simulink model "a01_SimTurret"  (R2024a)
settings: Solver=VariableStepAuto  StartTime=0.0  StopTime=10  FixedStep=0.000001  MaxStep=mSim.dTime*0.01  RelTol=mSim.dTime*0.01
PostLoadFcn:
  | a02_SimVariable
undefined symbols (not defined in the file): A02MTRPA, a1st, B01SCHED, b5th, C01ISENS, c7th, CRX1, DC, E03LIM, H01MDE, H01TRT, Init, mDefine, Mech, mSim, MtrPar, Sim, SIM, SimMde
libraries: spsSeriesRLCBranchLib x17, simulink x8, spsCurrentMeasurementLib x7, spsIGBTDiodeLib x7, spsDiodeLib x6, spsControlledVoltageSourceLib x6, spsVoltageMeasurementLib x4, SignalEditorBlockLib x3, spsDCVoltageSourceLib x1, spspowerguiLib x1
(part 3 of 3)

== stateflow chart a01_SimTurret/ASW_Composition/Subsystem/Nftn_StateManagement/Chart_StateManagement ==
  state Normal
    entry:
    mSMDE_uFlagRestart = Cnst_u16False;
    during:
    Ftn_CalActAngle();
    state Ftn_CalActAngle [function]
      (default) -> (junction 265) : // Calculation Acture Angle
      (junction 265) -> (junction 326) : {
          | sTemp = single(mMTPST_i64TurretPst - mSMDE_i64PstOrigin);
          | sTemp = sTemp * sAngleTrGain;
          | }
      (junction 326) -> (junction 328) [order 1] : [sTemp > Cnst_sZero]
      (junction 326) -> (junction 329) [order 2] : {
          | sTemp = (sTemp - single(int16(sTemp * Cnst_sInv360) * Cnst_s360)) + Cnst_s360;
          | }
      (junction 328) -> (junction 331) : {
          | sTemp = sTemp - single(int16(sTemp * Cnst_sInv360) * Cnst_s360);
          | }
      (junction 331) -> (junction 329)
      (junction 329) -> (junction 314)
      (junction 314) -> (junction 315) [order 1] : [sTemp > Cnst_s360]
      (junction 314) -> (junction 319) [order 2]
      (junction 315) -> (junction 317) : {
          | sTemp = sTemp - Cnst_s360;
          | }
      (junction 319) -> (junction 321) [order 1] : [sTemp < Cnst_sZero]
      (junction 319) -> (junction 316) [order 2] : {
          | sTemp = sTemp;
          | }
      (junction 321) -> (junction 322) : {
          | sTemp = sTemp + Cnst_s360;
          | }
      (junction 322) -> (junction 316)
      (junction 317) -> (junction 322)
      (junction 316) -> (junction 346)
      (junction 346) -> (junction 347) [order 1] : [uTurretDirection == Cnst_u16True]
      (junction 346) -> (junction 348) [order 2] : {
          | mSMDE_sActAngle = sTemp;
          | }
      (junction 347) -> (junction 349) : {
          | mSMDE_sActAngle = Cnst_s360 - sTemp;
          | }
      (junction 349) -> (junction 348)
      (junction 348) -> (junction 1542)
      (junction 1542) -> (junction 1543) [order 1] : [mSMDE_sRefAngle < Cnst_sZero]
      (junction 1543) -> (junction 1545) : {
          | mSMDE_sRefAngleDisp = mSMDE_sRefAngle + Cnst_s360;
          | }
      (junction 1542) -> (junction 1544) [order 2] : {
          | mSMDE_sRefAngleDisp = mSMDE_sRefAngle;
          | }
      (junction 1545) -> (junction 1544)
      (junction 1544) -> (junction 1546)
    note: 현재 위치 계산
    state Ftn_CalRefAngle [function]
      (default) -> (junction 799) : // Calculation Reference Angle
      (junction 799) -> (junction 896) [order 1] : [(mSMDE_i64PstOrigin ~= 0)&&(mCRX_uRefPst >= Cnst_u16One)]
      (junction 896) -> (junction 897)
      (junction 799) -> (junction 805) [order 2] : {
          | // Index 0 is not a valid value, but if index 0 is received, it is configured to move to the origin.
          | mSMDE_sRefAngle = Cnst_sZero;
          | }
      (junction 897) -> (junction 800) [order 1] : [(mCRX_uStart == Cnst_u16True)&&(uStartZ == Cnst_u16False)]
      (junction 897) -> (junction 900) [order 2] : // No Action
      (junction 800) -> (junction 801) : {
          | uFlagJogMde = Cnst_u16False;
          | }
      (junction 801) -> (junction 802) [order 1] : [mCRX_uRefPst > u16NumOfTool]
      (junction 801) -> (junction 803) [order 2] : {
          | uRefPst = mCRX_uRefPst;
          | }
      (junction 802) -> (junction 804) : {
          | uRefPst = u16NumOfTool;
          | }
      (junction 804) -> (junction 803)
      (junction 803) -> (junction 806) : {
          | mSMDE_sRefAngle = (single(uRefPst - Cnst_u16One) * sAnglePerTool);
          | Ftn_CalRefPst();
          | }
      (junction 806) -> (junction 900)
      (junction 900) -> (junction 805)
      (junction 805) -> (junction 807) : {
          | uStartZ = mCRX_uStart;
          | }
    note: Start 신호 입력시 Ref Angle 계산
    state Ftn_CalRefPst [function]
      (default) -> (junction 1433) : // Calculation Angle Error
      (junction 1433) -> (junction 1434) : {
          | mSMDE_uMtrCtrlMde = Cnst_MtrCtrlMde32Pst;
          | mSMDE_sAngleErr = mSMDE_sRefAngle - mSMDE_sActAngle;
          | }
      (junction 1434) -> (junction 1435) [order 1] : [mSMDE_sAngleErr < Cnst_sZero]
      (junction 1434) -> (junction 1436) [order 2] : {
          | sAbsAngleErr = mSMDE_sAngleErr;
          | }
      (junction 1435) -> (junction 1437) : {
          | sAbsAngleErr = -mSMDE_sAngleErr;
          | }
      (junction 1437) -> (junction 1436)
      (junction 1436) -> (junction 1438)
      (junction 1438) -> (junction 1439) [order 1] : // 각도 지령이 179~180도일 경우 또는 엔코더 포화시 근거리 운전 모드 -> 초기 멀티턴 방향으로 이동
          | [((sAbsAngleErr > Cnst_s179)&&(sAbsAngleErr < Cnst_s181))||((mSMDE_i64PstOrigin > i64EncMultiCtrlMax)&&(mSMDE_i64PstOrigin < (Cnst_i64EncMultiMax - i64EncMultiCtrlMax)))]
      (junction 1438) -> (junction 1440) [order 2]
      (junction 1439) -> (junction 1442)
      (junction 1440) -> (junction 1441) [order 1] : [mSMDE_sAngleErr > Cnst_s180]
      (junction 1442) -> (junction 1443) [order 1] : [uTurretDirection == Cnst_u16True]
      (junction 1440) -> (junction 1446) [order 2]
      (junction 1441) -> (junction 1467) : {
          | mSMDE_sRefAngle = mSMDE_sAngleErr - Cnst_s360;
          | }
      (junction 1442) -> (junction 1448) [order 2] : // uTurretDirection == Cnst_u16False
      (junction 1443) -> (junction 1444) : // uTurretDirection == Cnst_u16True
      (junction 1444) -> (junction 1445) [order 1] : [mSMDE_i64PstOrigin < i64EncMultiTurnOffset]
      (junction 1444) -> (junction 1450) [order 2] : // 멀티턴이 35535~65535 사이에 있을 경우 중앙(센터)에 가깝게 이동하기 위해 CW 방향으로 이동해야 함
      (junction 1445) -> (junction 1452) : // 멀티턴이 0~32768 사이에 있을 경우 중앙(센터)에 가깝게 이동하기 위해 CCW 방향으로 이동해야 함
      (junction 1446) -> (junction 1447) [order 1] : [mSMDE_sAngleErr < -Cnst_s180]
      (junction 1448) -> (junction 1449) [order 1] : [mSMDE_i64PstOrigin < i64EncMultiTurnOffset]
      (junction 1446) -> (junction 1465) [order 2] : {
          | mSMDE_sRefAngle = mSMDE_sAngleErr;
          | }
      (junction 1448) -> (junction 1454) [order 2] : // 멀티턴이 35535~65535 사이에 있을 경우 중앙(센터)에 가깝게 이동하기 위해 CW 방향으로 이동해야 함
      (junction 1449) -> (junction 1456) : // 멀티턴이 0~32768 사이에 있을 경우 중앙(센터)에 가깝게 이동하기 위해 CCW 방향으로 이동해야 함
      (junction 1447) -> (junction 1466) : {
          | mSMDE_sRefAngle = mSMDE_sAngleErr + Cnst_s360;
          | }
      (junction 1450) -> (junction 1451) [order 1] : [mSMDE_sAngleErr > Cnst_sZero]
      (junction 1452) -> (junction 1453) [order 1] : [mSMDE_sAngleErr > Cnst_sZero]
      (junction 1450) -> (junction 1464) [order 2] : {
          | // CCW 방향의 각도 지령일 경우  CCW 방향으로 이동(-180+360=180)
          | mSMDE_sRefAngle = mSMDE_sAngleErr;
          | }
      (junction 1451) -> (junction 1458) : {
          | // CW 방향의 각도 지령일 경우  CW 방향으로 이동(180=180)
          | mSMDE_sRefAngle = mSMDE_sAngleErr - Cnst_s360;
          | }
      (junction 1452) -> (junction 1459) [order 2] : {
          | // CCW 방향의 각도 지령일 경우  CCW 방향으로 이동(-180=-180)
          | mSMDE_sRefAngle = mSMDE_sAngleErr + Cnst_s360;
          | }
      (junction 1453) -> (junction 1460) : {
          | // CW 방향의 각도 지령일 경우  CCW 방향으로 이동(180-360=-180)
          | mSMDE_sRefAngle = mSMDE_sAngleErr;
          | }
      (junction 1454) -> (junction 1455) [order 1] : [mSMDE_sAngleErr > Cnst_sZero]
      (junction 1456) -> (junction 1457) [order 1] : [mSMDE_sAngleErr > Cnst_sZero]
      (junction 1454) -> (junction 1468) [order 2] : {
          | // CCW 방향의 각도 지령일 경우  CCW 방향으로 이동(-180+360=180)
          | mSMDE_sRefAngle = mSMDE_sAngleErr + Cnst_s360;
          | }
      (junction 1455) -> (junction 1461) : {
          | // CW 방향의 각도 지령일 경우  CW 방향으로 이동(180=180)
          | mSMDE_sRefAngle = mSMDE_sAngleErr;
          | }
      (junction 1456) -> (junction 1462) [order 2] : {
          | // CCW 방향의 각도 지령일 경우  CCW 방향으로 이동(-180=-180)
          | mSMDE_sRefAngle = mSMDE_sAngleErr;
          | }
      (junction 1457) -> (junction 1463) : {
          | // CW 방향의 각도 지령일 경우  CCW 방향으로 이동(180-360=-180)
          | mSMDE_sRefAngle = mSMDE_sAngleErr - Cnst_s360;
          | }
      (junction 1459) -> (junction 1458)
      (junction 1460) -> (junction 1459)
      (junction 1458) -> (junction 1464)
      (junction 1462) -> (junction 1461)
      (junction 1463) -> (junction 1462)
      (junction 1464) -> (junction 1463)
      (junction 1461) -> (junction 1468)
      (junction 1466) -> (junction 1465)
      (junction 1467) -> (junction 1466)
      (junction 1468) -> (junction 1467)
      (junction 1465) -> (junction 1469)
      (junction 1469) -> (junction 1470) [order 1] : [uTurretDirection == Cnst_u16True]
      (junction 1469) -> (junction 1471) [order 2] : {
          | mSMDE_i64PstRef = mMTPST_i64TurretPst + int64(single(i32BitPerRev) * (mSMDE_sRefAngle * Cnst_sInv360));
          | }
      (junction 1470) -> (junction 1472) : {
          | mSMDE_i64PstRef = mMTPST_i64TurretPst - int64(single(i32BitPerRev) * (mSMDE_sRefAngle * Cnst_sInv360));
          | }
      (junction 1472) -> (junction 1471)
      (junction 1471) -> (junction 1473)
    note: Ref Angle 재 계산 (가까운 목표 위치)
    state Ftn_CalExOutPst [function]
      note: uNumTool = (Deg / sAnglePerTool) + 1 +0.05;  // 소수 2째자리 반올림 0.05 반영
          | uNumTool = (Deg * sInvAnglePerTool) + 1 +0.05;
          | uNumTool = ((Deg * sInvAnglePerTool) + 1 +0.05) * 10;    // x10
          | uNumTool = single(int16(((Deg * sInvAnglePerTool) + 1 +0.05) * 10)) * 0.1;    // 소숫점이하 버림
          |
          | if(int16(uNumTool) == uNumTool)           // 정수 구하기
          | {
          | 	out = uint16(uNumTool);
          | }
      note: ▶ 현재 위치를 외부 24 V 신호로 출력
      (default) -> (junction 820) : // Calculating the Current Position and Setting the Digital Output
      (junction 820) -> (junction 821) : {
          | sNumTool = single(int16(((mSMDE_sActAngle * sInvAnglePerTool) + 1.0 + 0.05) * 10)) * 0.1;    // 소숫점이하 버림
          | }
      (junction 821) -> (junction 822) [order 1] : [mSMDE_sActAngle > (Cnst_s360 - sSetInPstAngleErr)]
      (junction 821) -> (junction 823) [order 2]
      (junction 822) -> (junction 825) : {
          | mSMDE_uExOut.uActPst = Cnst_u16One;
          | }
      (junction 823) -> (junction 824) [order 1] : [single(int16(sNumTool)*10.0) == (sNumTool*10.0)]
      (junction 823) -> (junction 826) [order 2] : {
          | mSMDE_uExOut.uActPst = Cnst_u16Zero;
          | }
      (junction 824) -> (junction 827) : {
          | mSMDE_uExOut.uActPst = uint16(sNumTool);
          | }
      (junction 825) -> (junction 827)
      (junction 827) -> (junction 826)
      (junction 826) -> (junction 828)
    state OriginDogin
      entry:
      mSMDE_uOprState = Cnst_OprMde32Origin;
      during:
      Ftn_OriginDogin();
      exit:
      mSMDE_uFlagSaveEncOrigin = Cnst_u16False;
      state Ftn_OriginDogin [function]
        (default) -> (junction 299) : {
            | mSMDE_uFlagInverterOut = Cnst_u16False;
            | }
        (junction 299) -> (junction 301) [order 1] : [(mCRX_uOrgin == Cnst_u16True)&&(mCRX_uDogin == Cnst_u16True)]
        (junction 299) -> (junction 96) [order 2]
        (junction 301) -> (junction 303) : // No Action
        (junction 96) -> (junction 115) [order 1] : [mCRX_uOrgin == Cnst_u16True]
        (junction 96) -> (junction 291) [order 2]
        (junction 115) -> (junction 112) : {
            | // Act uOrigin
            | mSMDE_uFlagSaveEncOrigin = Cnst_u16True;
            | mSMDE_sRefAngle = Cnst_sZero;
            | mSMDE_i64PstOrigin = mMTPST_i64TurretPst;
            | mSMDE_uExOut.uOrgNotDef = Cnst_u16False;
            | }
        (junction 291) -> (junction 293) [order 1] : [mCRX_uDogin == Cnst_u16True]
        (junction 291) -> (junction 117) [order 2] : // No Action
        (junction 293) -> (junction 294) : {
            | // Act uDogin
            | mSMDE_uFlagResetEnc = Cnst_u16True;
            | mSMDE_i64PstOrigin = 0;
            | mSMDE_uExOut.uOrgNotDef = Cnst_u16True;
            | }
        (junction 294) -> (junction 117)
        (junction 112) -> (junction 294)
        (junction 303) -> (junction 112)
        (junction 117) -> (junction 118) : {
            | mSMDE_i64PstRef = 0;
            | uOrginZ = mCRX_uOrgin;
            | uDoginZ = mCRX_uDogin;
            | uFlagResetEncZ = mI2c_uFlagResetEnc;
            | uFlagSaveEncOriginZ = mI2c_uFlagSaveEncOrigin;
            | }
    state Standby
      entry:
      mSMDE_uOprState = Cnst_OprMde1Standby;
      uFlagCmpltOpMde = Cnst_u16False;
      during:
      mSMDE_i64PstRef = mMTPST_i64TurretPst;
      mSMDE_i64PstRef = 0;
      uFlagCmpltOpMde = Cnst_u16False;
      mSMDE_sSpdLimit = sOprMdeSpdLim;
      Ftn_Standby();
      state Ftn_Standby [function]
        (default) -> (junction 62) : // Operation mode set (0: I/O, 1: Communication)
        (junction 62) -> (junction 65) [order 1] : [mCRX1_uRxChSel == Cnst_u16True]
        (junction 62) -> (junction 61) [order 2] : {
            | // I/O Operation
            | mSMDE_uFlagInverterOut = Cnst_u16False;
            | mSMDE_uMtrCtrlMde = Cnst_u16Zero;
            | mSMDE_sSpdRef = Cnst_sZero;
            | }
        (junction 65) -> (junction 63) : {
            | // CAN Operation
            | mSMDE_uFlagInverterOut = mCRX_uAllowingOperation;
            | mSMDE_uMtrCtrlMde = mCRX_uMtrCtrlMde;
            | mSMDE_sSpdRef = mCRX_sSpdCmd;
            | }
        (junction 63) -> (junction 61)
        (junction 61) -> (junction 64) : {
            | mSMDE_sSpdRefInSeqOut = mCTRL_sSpdRefIn;
            | mSMDE_sIfFreqSeqOut = mCTRL_sIfFreq;
            | uOrginZ = mCRX_uOrgin;
            | uDoginZ = mCRX_uDogin;
            | uFlagResetEncZ = mI2c_uFlagResetEnc;
            | uFlagSaveEncOriginZ = mI2c_uFlagSaveEncOrigin;
            | }
    state MpgJOG
      during:
      mSMDE_uFlagInverterOut = mCRX_uSvOn;
      Ftn_CalExOutPst();
      Ftn_MpgJogMde();
      %mSMDE_sSpdRefInSeqOut = mCTRL_sSpdRefIn;
      state Ftn_MpgJogMde [function]
        (default) -> (junction 859)
        (junction 859) -> (junction 136) : // Activation Mpg Jog Mode
            | {
            | mSMDE_uOprState = Cnst_OprMde4Mpg;
            | }
        (junction 136) -> (junction 137) [order 1] : [(mCRX_uPJog == Cnst_u16True)&&(mCRX_uNJog == Cnst_u16True)]
        (junction 136) -> (junction 841) [order 2] : {
            | mSMDE_i64PstRef = mMTPST_i64TurretPst;
            | mSMDE_uMtrCtrlMde = Cnst_MtrCtrlMde16Spd;
            | }
        (junction 137) -> (junction 139) : {
            | mSMDE_uMtrCtrlMde = Cnst_MtrCtrlMde32Pst;
            | mSMDE_sSpdRef = Cnst_sZero;
            | }
        (junction 841) -> (junction 843) [order 1] : [mCRX_uPJog == Cnst_u16True]
        (junction 843) -> (junction 844) : {
            | mSMDE_sSpdRef = -sMpgJogMdeSpdLim;
            | }
        (junction 841) -> (junction 1088) [order 2]
        (junction 1088) -> (junction 1090) [order 1] : [mCRX_uNJog == Cnst_u16True]
        (junction 1088) -> (junction 138) [order 2] : {
            | mSMDE_sSpdRef = Cnst_sZero;
            | }
        (junction 1090) -> (junction 1091) : {
            | mSMDE_sSpdRef = sMpgJogMdeSpdLim;
            | }
        (junction 1091) -> (junction 138)
        (junction 844) -> (junction 1091)
        (junction 139) -> (junction 844)
        (junction 138) -> (junction 857) : {
            | Ftn_CalRefAngle();
            | }
    state OperNJog
      entry:
      i32CntSenless = 0;
      // mSMDE_i64PstRef = mMTPST_i64TurretPst;
      during:
      mSMDE_uFlagInverterOut = mCRX_uSvOn;
      Ftn_MoveToRefPst();
      Ftn_CalAngleError();
      Ftn_CalExOutPst();
      // mSMDE_sSpdRefInSeqOut = mCTRL_sSpdRefIn;
      state Ftn_MoveToRefPst [function]
        (default) -> (junction 1097)
        (junction 1097) -> (junction 1098) [order 1] : [((mCRX_uPJog == Cnst_u16True)&&(mCRX_uNJog == Cnst_u16True))||((mCRX_uPJog == Cnst_u16False)&&(mCRX_uNJog == Cnst_u16False))]
        (junction 1097) -> (junction 1099) [order 2] : // Activation Jog Mode
            | {
            | mSMDE_uOprState = Cnst_OprMde2Jog;
            | mSMDE_uMtrCtrlMde = Cnst_MtrCtrlMde16Spd;
            | uFlagStepJogMde = Cnst_u16True;
            | uFlagJogMde = Cnst_u16True;
            | }
        (junction 1098) -> (junction 1101) : {
            | mSMDE_uOprState = Cnst_OprMde8Operation;
            | mSMDE_uMtrCtrlMde = Cnst_MtrCtrlMde32Pst;
            | }
        (junction 1099) -> (junction 1100) [order 1] : [mCRX_uPJog == Cnst_u16True]
        (junction 1101) -> (junction 1102) [order 1] : [uFlagStepJogMde == Cnst_u16True]
        (junction 1101) -> (junction 1533) [order 2] : {
            | mSMDE_sSpdLimit = sOprMdeSpdLim;
            | }
        (junction 1102) -> (junction 1118) : {
            | mSMDE_sSpdLimit = sJogMdeSpdRLim;
            | uFlagStepJogMde = Cnst_u16False;
            | Ftn_CalRefAngle();
            | }
        (junction 1099) -> (junction 1103) [order 2]
        (junction 1100) -> (junction 1105)
        (junction 1103) -> (junction 1104) [order 1] : [uFalg_PJog_Step == Cnst_u16False]
        (junction 1105) -> (junction 1106) [order 1] : [uFalg_NJog_Step == Cnst_u16False]
        (junction 1104) -> (junction 1428) : {
            | uFalg_NJog_Step = Cnst_u16True;
            | mSMDE_sSpdRef = -sJogMdeSpdRLim;
            | }
        (junction 1106) -> (junction 1154) : {
            | uFalg_PJog_Step = Cnst_u16True;
            | mSMDE_sSpdRef = -sJogMdeSpdRLim;
            | }
        (junction 1103) -> (junction 1112) [order 2] : // No Action
        (junction 1105) -> (junction 1114) [order 2] : // No Action
        (junction 1118) -> (junction 1533)
        (junction 1533) -> (junction 1115) : {
            | Ftn_CalRefAngle();
            | }
        (junction 1428) -> (junction 1421) [order 1] : [uTurretDirection == Cnst_u16True]
        (junction 1154) -> (junction 1156) [order 1] : [uTurretDirection == Cnst_u16True]
        (junction 1428) -> (junction 1422) [order 2] : {
            | uNexRefPst = uint16(sNumTool + Cnst_sHalf);
            | mSMDE_sRefAngle = (single(uNexRefPst + Cnst_u16One) * sAnglePerTool);
            | }
        (junction 1421) -> (junction 1426) : {
            | uNexRefPst = uint16(sNumTool - Cnst_sHalf);
            | mSMDE_sRefAngle = (single(uNexRefPst - Cnst_u16One) * sAnglePerTool);
            | }
        (junction 1154) -> (junction 1111) [order 2] : {
            | uNexRefPst = uint16(sNumTool - Cnst_sHalf);
            | mSMDE_sRefAngle = (single(uNexRefPst - Cnst_u16One) * sAnglePerTool);
            | }
        (junction 1156) -> (junction 1157) : {
            | uNexRefPst = uint16(sNumTool + Cnst_sHalf);
            | mSMDE_sRefAngle = (single(uNexRefPst + Cnst_u16One) * sAnglePerTool);
            | }
        (junction 1422) -> (junction 1112)
        (junction 1426) -> (junction 1422)
        (junction 1114) -> (junction 1426)
        (junction 1111) -> (junction 1114)
        (junction 1157) -> (junction 1111)
        (junction 1115) -> (junction 1157)
        (junction 1112) -> (junction 1119)
      state Ftn_CalAngleError [function]
        (default) -> (junction 761) : // Calculation Angle Error
        (junction 761) -> (junction 1554) : {
            | //mSMDE_uMtrCtrlMde = Cnst_MtrCtrlMde32Pst;
            | mSMDE_sAngleErr = mSMDE_sRefAngle - mSMDE_sActAngle;
            | }
        (junction 1554) -> (junction 1555) [order 1] : [mSMDE_sAngleErr < Cnst_s180]
        (junction 1554) -> (junction 1556) [order 2] : // No Action
        (junction 1555) -> (junction 1557) : {
            | mSMDE_sAngleErr = mSMDE_sAngleErr + Cnst_s360;
            | }
        (junction 1557) -> (junction 1556)
        (junction 1556) -> (junction 762)
        (junction 762) -> (junction 763) [order 1] : [mSMDE_sAngleErr < Cnst_sZero]
        (junction 762) -> (junction 764) [order 2] : {
            | sAbsAngleErr = mSMDE_sAngleErr;
            | }
        (junction 763) -> (junction 765) : {
            | sAbsAngleErr = -mSMDE_sAngleErr;
            | }
        (junction 765) -> (junction 764)
        (junction 764) -> (junction 766)
        (junction 766) -> (junction 767) [order 1] : [(sAbsAngleErr < sSetInPstAngleErr)||(sAbsAngleErr > Cnst_s360 - sSetInPstAngleErr)]
        (junction 766) -> (junction 772) [order 2] : {
            | mSMDE_uExOut.uInPst = Cnst_u16False;
            | i32CntSenless = 0;
            | }
        (junction 767) -> (junction 768)
        (junction 768) -> (junction 769) [order 1] : [i32CntSenless >= i32CntSetInPst]
        (junction 768) -> (junction 773) [order 2] : {
            | i32CntSenless++;
            | }
        (junction 769) -> (junction 770) : {
            | i32CntSenless = i32CntSetInPst;
            | mSMDE_uExOut.uInPst = Cnst_u16True;
            | }
        (junction 770) -> (junction 771) [order 1] : [mCRX_uStop == Cnst_u16True]
        (junction 770) -> (junction 774) [order 2] : // No Action
        (junction 771) -> (junction 775) : {
            | mSMDE_uFlagInverterOut = Cnst_u16False;
            | uFlagCmpltOpMde = Cnst_u16True;
            | i32CntSenless = 0;
            | }
        (junction 773) -> (junction 772)
        (junction 774) -> (junction 773)
        (junction 775) -> (junction 774)
        (junction 772) -> (junction 776)
    (default) -> Standby
    Standby -> OriginDogin [order 1] : [((mCRX_uOrgin == Cnst_u16True)&&(uOrginZ == Cnst_u16False))||((mCRX_uDogin == Cnst_u16True)&&(uDoginZ == Cnst_u16False))]
    OriginDogin -> Standby [order 1] : [(mI2c_uFlagResetEnc == Cnst_u16False)&&(uFlagResetEncZ == Cnst_u16True)]
    OriginDogin -> Standby [order 2] : [(mI2c_uFlagSaveEncOrigin == Cnst_u16False)&&(uFlagSaveEncOriginZ == Cnst_u16True)]
    Standby -> MpgJOG [order 2] : [(mCRX_uSvOn == Cnst_u16True)&&(mCRX_uEnMpg == Cnst_u16True)]
    MpgJOG -> Standby : [mCRX_uSvOn == Cnst_u16False]
    OperNJog -> MpgJOG [order 2] : [(mCRX_uSvOn == Cnst_u16True)&&(mCRX_uEnMpg == Cnst_u16True)]
    Standby -> OperNJog [order 3] : [(mCRX_uSvOn == Cnst_u16True)&&(mSMDE_i64PstOrigin ~= 0)&&((mCRX_uPJog == Cnst_u16True)||(mCRX_uNJog == Cnst_u16True))]
    Standby -> OperNJog [order 4] : [(mCRX_uSvOn == Cnst_u16True)&&(mSMDE_i64PstOrigin ~= 0)&&(mCRX_uStart == Cnst_u16True)&&(uStartZ == Cnst_u16False)]
    OperNJog -> Standby [order 1] : [(mCRX_uSvOn == Cnst_u16False)||(uFlagCmpltOpMde == Cnst_u16True)]
  state Wait
    entry:
    mSMDE_uOprState = Cnst_OprMde16Wait;
    mSMDE_uFlagRestart = Cnst_u16False;
    i32CntSenless = 0;
    during:
    Ftn_Wait();
    state Ftn_Wait [function]
      (default) -> (junction 250) : {
          | mSMDE_uFlagInverterOut = Cnst_u16False;
          | }
      (junction 250) -> (junction 251) [order 1] : [i32CntSenless >= i32CntSetRdyRestart]
      (junction 250) -> (junction 252) [order 2] : {
          | i32CntSenless++;
          | }
      (junction 251) -> (junction 253) : {
          | i32CntSenless = i32CntSetRdyRestart;
          | mSMDE_uFlagRestart = Cnst_u16True;
          | }
      (junction 253) -> (junction 252)
      (junction 252) -> (junction 254)
  (default) -> Normal
  Normal -> Wait : [mDIAG_uFltStat == Cnst_u16True]
  Wait -> Normal : [(mDIAG_uFltStat == Cnst_u16False)&&(mSMDE_uFlagRestart == Cnst_u16True)]
  data: mCRX1_uRxChSel input; mCRX_uAllowingOperation input; mCRX_uMtrCtrlMde input; mCRX_sSpdCmd input; mCRX_uOrgin input; mCRX_uDogin input; mCRX_uEnMpg input; mCRX_uPJog input; mCRX_uNJog input; mCRX_uRefPst input; mCRX_uSvOn input; mCRX_uStop input; mCRX_uStart input; mCTRL_sSpdRefIn input; mCTRL_sIfFreq input; mSMDE_uFlagInverterOut output uint16; mSMDE_uMtrCtrlMde output uint16; mSMDE_sSpdRef output single; mSMDE_sSpdLimit output single; mSMDE_sSpdRefInSeqOut output single; mSMDE_sIfFreqSeqOut output single; Cnst_u16False constant uint16 =CnstNr.C_u16_0; Cnst_u16Zero constant uint16 =CnstNr.C_u16_0; Cnst_sZero constant single =CnstNr.C_sZero; mSMDE_uOprState output uint16; mSMDE_uFlagSaveEncOrigin output uint16; mSMDE_uFlagResetEnc output uint16; mSMDE_i64PstOrigin output int64 =4294180863; Cnst_OprMde1Standby constant uint16 =1; Cnst_OprMde32Origin constant uint16 =32; Cnst_u16True constant uint16 =CnstNr.C_u16_1; mI2c_uFlagSaveEncOrigin input; mI2c_uFlagResetEnc input; mSMDE_i64PstRef output int64; mSMDE_uExOut output Bus: X_H01EXO; Cnst_OprMde4Mpg constant uint16 =4; mMTPST_i64TurretPst input; mDIAG_uFltStat input; uTurretDirection input; u16NumOfTool input; sSetInPstAngleErr input; mSMDE_sRefAngle output single; mSMDE_sRefAngleDisp output single; mSMDE_sActAngle output single; mSMDE_sAngleErr output single; sAnglePerTool input; sAngleTrGain input; Cnst_u16One constant uint16 =CnstNr.C_u16_1; uRefPst local uint16; Cnst_OprMde16Wait constant uint16 =16; mSMDE_uFlagRestart output uint16; i32CntSenless output int32; i32CntSetRdyRestart input; uDoginZ local uint16; uOrginZ local uint16; uFlagResetEncZ output uint16; uFlagSaveEncOriginZ output uint16; Cnst_s360 constant single =360; Cnst_sInv360 constant single =1/360; sTemp local single; Cnst_OprMde8Operation constant uint16 =8; sAbsAngleErr local single; i32CntSetInPst input; sInvAnglePerTool input; sOprMdeSpdLim input; uFlagCmpltOpMde local uint16; Cnst_MtrCtrlMde16Spd constant uint16 =CnstMde.C_MODE16_SPD; sJogMdeSpdRLim input; Cnst_MtrCtrlMde32Pst constant uint16 =CnstMde.C_MODE32_PST; Cnst_OprMde2Jog constant uint16 =2; sMpgJogMdeSpdLim input; uFalg_NJog_Step local uint16; uFalg_PJog_Step local uint16; Cnst_s179 constant single =179; Cnst_s181 constant single =181; i64EncMultiCtrlMax input; Cnst_i64EncMultiMax constant int64 =65535; i64EncMultiTurnOffset input; Cnst_s180 constant single =180; i32BitPerRev input; uFlagJogMde local uint16; uFlagStepJogMde local uint16; sNumTool output single; Cnst_sHalf constant single =0.5; uNexRefPst local uint16; uStartZ local uint16

== stateflow chart a01_SimTurret/BSW_CAN/Data_Interation1 ==
  (default) -> (junction 86)
  (junction 86) -> (junction 11) : {
      | u32Tx_Data = uint32((a18sCanRxMaster[i32CntArrNo] - a18sOffset[i32CntArrNo]) * a18sInvFactor[i32CntArrNo]);
      | }
  (junction 11) -> (junction 118) [order 1] : [a18u32StartBit[i32CntArrNo] >= 32]
  (junction 11) -> (junction 114) [order 2] : {
      | a18u32High[i32CntArrNo] = 0;
      | }
  (junction 118) -> (junction 127) : {
      | a18u32Low[i32CntArrNo] = 0;
      | }
  (junction 127) -> (junction 122) [order 1] : [a18u32StartBit[i32CntArrNo] == 32]
  (junction 114) -> (junction 45) [order 1] : [a18u32StartBit[i32CntArrNo] > 0]
  (junction 127) -> (junction 123) [order 2] : {
      | a18u32High[i32CntArrNo] = uint32(u32Tx_Data<<(a18u32StartBit[i32CntArrNo]-32));
      | }
  (junction 122) -> (junction 135) : {
      | a18u32High[i32CntArrNo] = u32Tx_Data;
      | }
  (junction 114) -> (junction 38) [order 2] : {
      | a18u32Low[i32CntArrNo] = u32Tx_Data;
      | }
  (junction 45) -> (junction 46) : {
      | a18u32Low[i32CntArrNo] = uint32(u32Tx_Data<<a18u32StartBit[i32CntArrNo]);
      | }
  (junction 46) -> (junction 38)
  (junction 135) -> (junction 123)
  (junction 38) -> (junction 141) : {
      | mCRX1_u32CrrDataLow = mCRX1_u32CrrDataLow & a18sClearBitRx1[i32CntArrNo];
      | mCRX1_u32CrrDataLow = mCRX1_u32CrrDataLow | a18u32Low[i32CntArrNo];
      | }
  (junction 123) -> (junction 151) : {
      | mCRX1_u32CrrDataHigh = mCRX1_u32CrrDataHigh & a18sClearBitRx1[i32CntArrNo];
      | mCRX1_u32CrrDataHigh = mCRX1_u32CrrDataHigh | a18u32High[i32CntArrNo];
      | }
  (junction 151) -> (junction 141)
  (junction 141) -> (junction 14)
  data: a18sCanRxMaster input single size=18; a18u32StartBit input size=18; a18sInvFactor input size=18; a18sOffset input size=18; a18sClearBitRx1 input size=18; a18u32Low output uint32 size=18; a18u32High output uint32 size=18; mCRX1_u32CrrDataLow output uint32; u32Tx_Data local uint32 size=1; i32CntArrNo input size=1; mCRX1_u32CrrDataHigh output uint32 =33488896
